simulink model "observadores_simulink"  (R2025b)
settings: Solver=VariableStepAuto  StartTime=0.0  StopTime=10.0  RelTol=1e-3
values from neighbouring files (symbols this model uses):
  A = [0 1;-2 -3 ]    [observadores.m]
  B = [0;1]    [observadores.m]
  C = [1 0]    [observadores.m]
  D = 0    [observadores.m]
  x1 = [0;0]    [observadores.m]
libraries: eeLuenbergerObserver x1
settings Model: Creator=Froilán Pardo  LastModifiedBy=Froilán Pardo

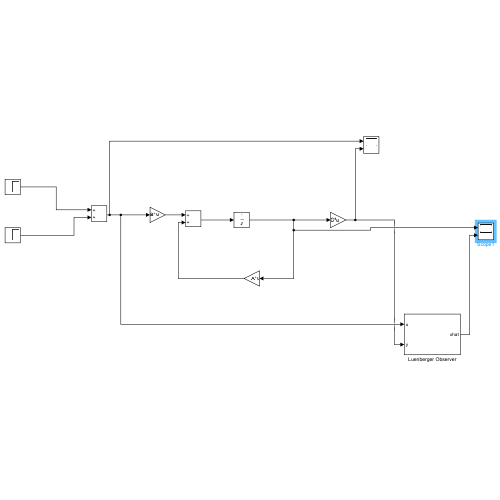
[thumbnail: Simulink's stored preview of the top-level diagram]
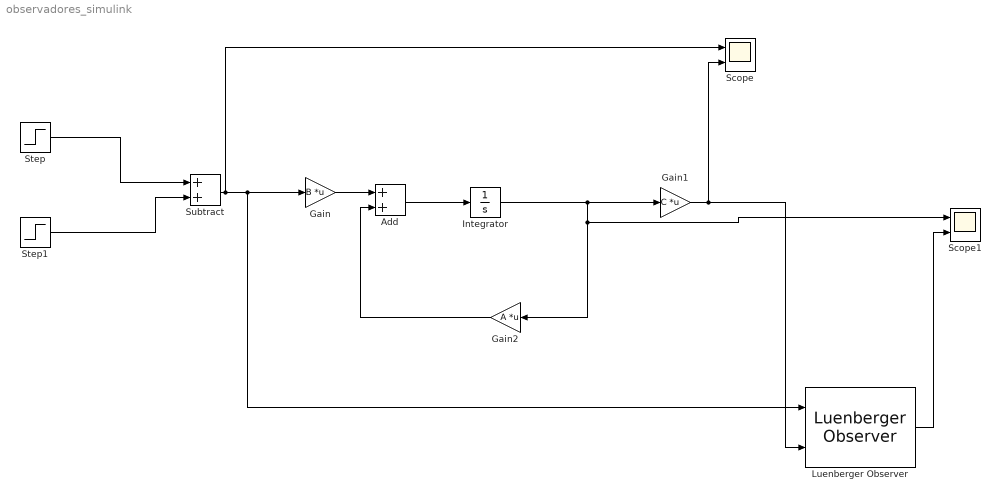
== system observadores_simulink ==
  Add : Sum
  Gain : Gain  Gain=B  Multiplication=Matrix(K*u)
  Gain1 : Gain  Gain=C  Multiplication=Matrix(K*u)
  Gain2 : Gain  Gain=A  Multiplication=Matrix(K*u)
  Integrator : Integrator  InitialCondition=x1
  Luenberger Observer : eeLuenbergerObserver/Luenberger Observer  StateSpaceType=Continuous-time  Ad=1  Bd=1  Cd=1  Dd=1  A=A  B=B  C=C  D=D  ObserverDesign=Desired eigenvalues  Ld=1  DesiredEigenvalues=polos  x0=x0  Tsd=0.1  Ts=0.1
      settings: LibrarySourceBlock=ee_sl_lib/Observers/Luenberger Observer
  Scope : Scope  NumInputPorts=2
      settings: ActiveDisplayYMinimum=-1  ActiveDisplayYMaximum=1
  Scope1 : Scope  NumInputPorts=2
      settings: ActiveDisplayYMinimum=-0.24999999999999994  ActiveDisplayYMaximum=2.25
  Step : Step  SampleTime=0
  Step1 : Step  Time=5  SampleTime=0
  Subtract : Sum
  wires:
  Step1/1 -> Subtract/2
  Subtract/1 -> Luenberger Observer/1, Gain/1, Scope/1
  Gain2/1 -> Add/2
  Gain/1 -> Add/1
  Add/1 -> Integrator/1
  Integrator/1 -> Gain2/1, Scope1/1, Gain1/1
  Gain1/1 -> Scope/2, Luenberger Observer/2
  Luenberger Observer/1 -> Scope1/2
  Step/1 -> Subtract/1
